simulink model "TailSitter_PX4"  (R2018b)
settings: Solver=VariableStepAuto  StartTime=0.0  StopTime=1100  RelTol=1e-3
values from neighbouring files (symbols this model uses):
  p =     [ds.mat]    (also in vxs.mat)
undefined symbols (not defined in the file or in its folder): quatnormalize
libraries: aerolibutil x24, simulink x14, sharedtransform x6, vrlib x4, sharedutil x3, simulink_extras x2, aerolibanim x1, aerolibanimutils x1
(part 2 of 3)

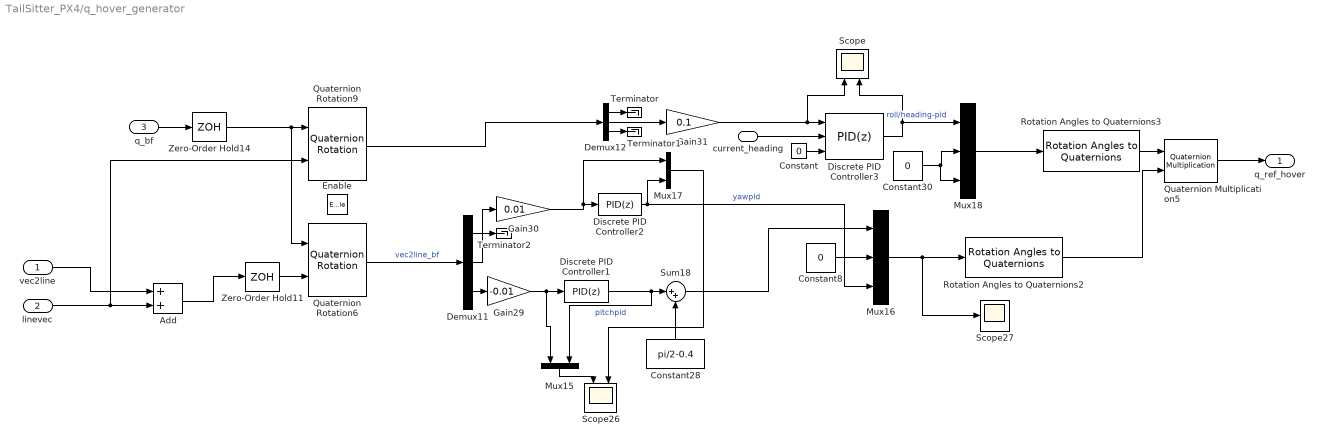
== system TailSitter_PX4/q_hover_generator ==
  vec2line : Inport
  linevec : Inport  Port=2
  q_bf : Inport  Port=3
  current_heading : Inport  Port=4
  Enable : EnablePort  StatesWhenEnabling=reset
  Add : Sum
  Constant : Constant  Value=0
  Constant28 : Constant  Value=pi/2-0.4
  Constant30 : Constant  Value=0
  Constant8 : Constant  Value=0
  Demux11 : Demux  Outputs=3
  Demux12 : Demux  Outputs=3
  Discrete PID Controller1 : simulink/Continuous/PID Controller  Controller=PID  Form=Parallel  TimeDomain=Discrete-time  SampleTime=-1  IntegratorMethod=Forward Euler  FilterMethod=Forward Euler  ControllerParametersSource=internal  P=0.75  I=0.1  D=8  UseFilter=off  N=100  TunerSelectOption=Transfer Function Based (PID Tuner App)  InitialConditionSource=internal  InitialConditionForIntegrator=0  InitialConditionForFilter=0  DifferentiatorICPrevScaledInput=0  ExternalReset=none  TrackingMode=off  Kt=1  LimitOutput=on  UpperSaturationLimit=deg2rad(40)  LowerSaturationLimit=-deg2rad(40)  LinearizeAsGain=off  AntiWindupMode=none  Kb=1  POutMin=[]  POutMax=[]  IOutMin=[]  IOutMax=[]  DOutMin=[]  DOutMax=[]  NOutMin=[]  NOutMax=[]  SumOutMin=[]  SumOutMax=[]  SaturationOutMin=[]  SaturationOutMax=[]  PParamMin=[]  PParamMax=[]  IParamMin=[]  IParamMax=[]  DParamMin=[]  DParamMax=[]  NParamMin=[]  NParamMax=[]  KbParamMin=[]  KbParamMax=[]  KtParamMin=[]  KtParamMax=[]  KbOutMin=[]  KbOutMax=[]  KtOutMin=[]  KtOutMax=[]  IntegratorOutMin=[]  IntegratorOutMax=[]  FilterOutMin=[]  FilterOutMax=[]  SumI1OutMin=[]  SumI1OutMax=[]  SumI2OutMin=[]  SumI2OutMax=[]  SumI3OutMin=[]  SumI3OutMax=[]  SumI4OutMin=[]  SumI4OutMax=[]  SumDOutMin=[]  SumDOutMax=[]  DifferentiatorOutMin=[]  DifferentiatorOutMax=[]  FilterDiffOutCoefMin=[]  FilterDiffOutCoefMax=[]  ReciprocalOutMin=[]  ReciprocalOutMax=[]  SumDenOutMin=[]  SumDenOutMax=[]  SumNumOutMin=[]  SumNumOutMax=[]  DivideOutMin=[]  DivideOutMax=[]  IntegratorContinuousStateAttributes=''  IntegratorStateMustResolveToSignalObject=off  IntegratorRTWStateStorageClass=Auto  FilterContinuousStateAttributes=''  FilterStateMustResolveToSignalObject=off  FilterRTWStateStorageClass=Auto  ParallelPVariant=InternalParameters  IdealPVariant=Disabled  IVariant=InternalParameters  DVariant=InternalParameters  IntegratorVariant=Discrete  SatVariant=Enabled  AWVariant=Passthrough  PCopyVariant=Disabled  TRVariant=Disabled  FdbkBlocksVariant=Forward  IdealPFdbkVariant=Disabled  SatFdbkVariant=Disabled  DerivativeFilterVariant=Differentiator  NVariant=Passthrough  NCopyVariant=Disabled_SignalSpec  FilterICVariant=InternalICsDifferentiator  IntegratorICVariant=InternalICs  ExternalResetVariant=Disabled  TRSumVariant=Passthrough  SumFdbkVariant=Disabled  SumVariant=Sum_PID
  Discrete PID Controller2 : simulink/Continuous/PID Controller  Controller=PID  Form=Parallel  TimeDomain=Discrete-time  SampleTime=-1  IntegratorMethod=Forward Euler  FilterMethod=Forward Euler  ControllerParametersSource=internal  P=1  I=0  D=2  UseFilter=off  N=100  TunerSelectOption=Transfer Function Based (PID Tuner App)  InitialConditionSource=internal  InitialConditionForIntegrator=0  InitialConditionForFilter=0  DifferentiatorICPrevScaledInput=0  ExternalReset=none  TrackingMode=off  Kt=1  LimitOutput=on  UpperSaturationLimit=deg2rad(40)  LowerSaturationLimit=-deg2rad(40)  LinearizeAsGain=off  AntiWindupMode=none  Kb=1  POutMin=[]  POutMax=[]  IOutMin=[]  IOutMax=[]  DOutMin=[]  DOutMax=[]  NOutMin=[]  NOutMax=[]  SumOutMin=[]  SumOutMax=[]  SaturationOutMin=[]  SaturationOutMax=[]  PParamMin=[]  PParamMax=[]  IParamMin=[]  IParamMax=[]  DParamMin=[]  DParamMax=[]  NParamMin=[]  NParamMax=[]  KbParamMin=[]  KbParamMax=[]  KtParamMin=[]  KtParamMax=[]  KbOutMin=[]  KbOutMax=[]  KtOutMin=[]  KtOutMax=[]  IntegratorOutMin=[]  IntegratorOutMax=[]  FilterOutMin=[]  FilterOutMax=[]  SumI1OutMin=[]  SumI1OutMax=[]  SumI2OutMin=[]  SumI2OutMax=[]  SumI3OutMin=[]  SumI3OutMax=[]  SumI4OutMin=[]  SumI4OutMax=[]  SumDOutMin=[]  SumDOutMax=[]  DifferentiatorOutMin=[]  DifferentiatorOutMax=[]  FilterDiffOutCoefMin=[]  FilterDiffOutCoefMax=[]  ReciprocalOutMin=[]  ReciprocalOutMax=[]  SumDenOutMin=[]  SumDenOutMax=[]  SumNumOutMin=[]  SumNumOutMax=[]  DivideOutMin=[]  DivideOutMax=[]  IntegratorContinuousStateAttributes=''  IntegratorStateMustResolveToSignalObject=off  IntegratorRTWStateStorageClass=Auto  FilterContinuousStateAttributes=''  FilterStateMustResolveToSignalObject=off  FilterRTWStateStorageClass=Auto  ParallelPVariant=InternalParameters  IdealPVariant=Disabled  IVariant=InternalParameters  DVariant=InternalParameters  IntegratorVariant=Discrete  SatVariant=Enabled  AWVariant=Passthrough  PCopyVariant=Disabled  TRVariant=Disabled  FdbkBlocksVariant=Forward  IdealPFdbkVariant=Disabled  SatFdbkVariant=Disabled  DerivativeFilterVariant=Differentiator  NVariant=Passthrough  NCopyVariant=Disabled_SignalSpec  FilterICVariant=InternalICsDifferentiator  IntegratorICVariant=InternalICs  ExternalResetVariant=Disabled  TRSumVariant=Passthrough  SumFdbkVariant=Disabled  SumVariant=Sum_PID
  Discrete PID Controller3 : simulink/Continuous/PID Controller  Controller=PID  Form=Parallel  TimeDomain=Discrete-time  SampleTime=-1  IntegratorMethod=Forward Euler  FilterMethod=Forward Euler  ControllerParametersSource=internal  P=1  I=1  D=0  UseFilter=off  N=100  TunerSelectOption=Transfer Function Based (PID Tuner App)  InitialConditionSource=external  InitialConditionForIntegrator=0  InitialConditionForFilter=0  DifferentiatorICPrevScaledInput=0  ExternalReset=none  TrackingMode=off  Kt=1  LimitOutput=off  UpperSaturationLimit=deg2rad(40)  LowerSaturationLimit=-deg2rad(40)  LinearizeAsGain=off  AntiWindupMode=none  Kb=1  POutMin=[]  POutMax=[]  IOutMin=[]  IOutMax=[]  DOutMin=[]  DOutMax=[]  NOutMin=[]  NOutMax=[]  SumOutMin=[]  SumOutMax=[]  SaturationOutMin=[]  SaturationOutMax=[]  PParamMin=[]  PParamMax=[]  IParamMin=[]  IParamMax=[]  DParamMin=[]  DParamMax=[]  NParamMin=[]  NParamMax=[]  KbParamMin=[]  KbParamMax=[]  KtParamMin=[]  KtParamMax=[]  KbOutMin=[]  KbOutMax=[]  KtOutMin=[]  KtOutMax=[]  IntegratorOutMin=[]  IntegratorOutMax=[]  FilterOutMin=[]  FilterOutMax=[]  SumI1OutMin=[]  SumI1OutMax=[]  SumI2OutMin=[]  SumI2OutMax=[]  SumI3OutMin=[]  SumI3OutMax=[]  SumI4OutMin=[]  SumI4OutMax=[]  SumDOutMin=[]  SumDOutMax=[]  DifferentiatorOutMin=[]  DifferentiatorOutMax=[]  FilterDiffOutCoefMin=[]  FilterDiffOutCoefMax=[]  ReciprocalOutMin=[]  ReciprocalOutMax=[]  SumDenOutMin=[]  SumDenOutMax=[]  SumNumOutMin=[]  SumNumOutMax=[]  DivideOutMin=[]  DivideOutMax=[]  IntegratorContinuousStateAttributes=''  IntegratorStateMustResolveToSignalObject=off  IntegratorRTWStateStorageClass=Auto  FilterContinuousStateAttributes=''  FilterStateMustResolveToSignalObject=off  FilterRTWStateStorageClass=Auto  ParallelPVariant=InternalParameters  IdealPVariant=Disabled  IVariant=InternalParameters  DVariant=InternalParameters  IntegratorVariant=Discrete  SatVariant=Disabled  AWVariant=Passthrough  PCopyVariant=Disabled  TRVariant=Disabled  FdbkBlocksVariant=Forward  IdealPFdbkVariant=Disabled  SatFdbkVariant=Disabled  DerivativeFilterVariant=Differentiator  NVariant=Passthrough  NCopyVariant=Disabled_SignalSpec  FilterICVariant=ExternalICs  IntegratorICVariant=ExternalICs  ExternalResetVariant=Disabled  TRSumVariant=Passthrough  SumFdbkVariant=Disabled  SumVariant=Sum_PID
  Gain29 : Gain  Gain=-0.01
  Gain30 : Gain  Gain=0.01
  Gain31 : Gain  Gain=0.1
  Mux15 : Mux  Inputs=2
  Mux16 : Mux  Inputs=3
  Mux17 : Mux  Inputs=2
  Mux18 : Mux  Inputs=3
  Quaternion Multiplication5 : aerolibutil/Quaternion Multiplication
  Quaternion Rotation6 : aerolibutil/Quaternion Rotation
  Quaternion Rotation9 : aerolibutil/Quaternion Rotation
  Rotation Angles to Quaternions2 : sharedtransform/Rotation Angles to Quaternions  rotationOrder=YXZ  aMode=aMode
      settings: SourceProductName=Aerospace Blockset  SourceProductBaseCode=AE
  Rotation Angles to Quaternions3 : sharedtransform/Rotation Angles to Quaternions  rotationOrder=ZYX  aMode=aMode
      settings: SourceProductName=Aerospace Blockset  SourceProductBaseCode=AE
  Scope : Scope  NumInputPorts=2
  Scope26 : Scope  NumInputPorts=2
  Scope27 : Scope
  Sum18 : Sum  Inputs=|++
  Terminator : Terminator
  Terminator1 : Terminator
  Terminator2 : Terminator
  Zero-Order Hold11 : ZeroOrderHold  SampleTime=p.Ts
  Zero-Order Hold14 : ZeroOrderHold  SampleTime=p.Ts
  q_ref_hover : Outport
  wires:
  vec2line/1 -> Add/1
  Discrete PID Controller1/1 -> Sum18/1, Mux15/2  "pitchpid"
  Gain29/1 -> Mux15/1, Discrete PID Controller1/1
  Demux11/2 -> Gain30/1
  Quaternion Rotation6/1 -> Demux11/1  "vec2line_bf"
  Constant30/1 -> Mux18/3, Mux18/2
  Demux12/3 -> Terminator1/1
  Demux12/1 -> Terminator/1
  Gain31/1 -> Scope/1, Discrete PID Controller3/1
  linevec/1 -> Quaternion Rotation9/2, Add/2
  Discrete PID Controller3/1 -> Scope/2, Mux18/1  "roll/heading-pid"
  Mux15/1 -> Scope26/1
  Mux16/1 -> Scope27/1, Rotation Angles to Quaternions2/1
  Rotation Angles to Quaternions3/1 -> Quaternion Multiplication5/1
  q_bf/1 -> Zero-Order Hold14/1
  Demux11/3 -> Gain29/1
  Constant8/1 -> Mux16/2
  Discrete PID Controller2/1 -> Mux16/3, Mux17/2  "yawpid"
  Rotation Angles to Quaternions2/1 -> Quaternion Multiplication5/2
  Mux18/1 -> Rotation Angles to Quaternions3/1
  Quaternion Multiplication5/1 -> q_ref_hover/1
  Demux12/2 -> Gain31/1
  Mux17/1 -> Scope26/2
  Add/1 -> Zero-Order Hold11/1
  Zero-Order Hold14/1 -> Quaternion Rotation6/1, Quaternion Rotation9/1
  Constant28/1 -> Sum18/2
  Gain30/1 -> Mux17/1, Discrete PID Controller2/1
  Zero-Order Hold11/1 -> Quaternion Rotation6/2
  Demux11/1 -> Terminator2/1
  Sum18/1 -> Mux16/1
  Constant/1 -> Discrete PID Controller3/3
  current_heading/1 -> Discrete PID Controller3/2
  Quaternion Rotation9/1 -> Demux12/1

== matlab function TailSitter_PX4/Torque_FL ==
  data: u_omegaL output; u_omegaR output; u_deltaL output; u_deltaR output; tao input; states input; u_jointT input; p parameter
function [u_omegaL,u_omegaR, u_deltaL,u_deltaR]  = FL_torques(tao, states, u_jointT, p)


wxr = tao(1); % I wonder if this comversion from omega to tao is right? Depends on Emil Fresk implementation
wyr = tao(2);
wzr = tao(3);
v = states(1:3);
vx = v(1);
vy = v(2);
vz = v(3);
w = states(4:6);
wx = w(1);
wy = w(2);
wz = w(3);
q = states(7:10); % Possibly not needed?
q0=q(1);
q1=q(2);
q2=q(3);
q3=(4);
deltaL = states(11);
deltaR = states(12);
omegaL = states(13);
omegaR = states(14);

% init output vector
u_deltaL = 0;
u_deltaR = 0;
u_omegaL = 0;
u_omegaR = 0;

% If you know of a better way (not counting modifying the code below to use
% p.x notation, plese feel welcome to tell me.
%P = struct2cell(p);
%Pn = fieldnames(p);
%for i=1:numel(P)
%    eval(Pn{i}+"="+string(P{i})+";")
%end
Ts=p.Ts;
m=p.m;
Ix=p.Ix;
Iy=p.Iy;
Iz=p.Iz;
I=p.I;
g=p.g;
rho=p.rho;
propd=p.propd;
K_T=p.K_T;
K_v=p.K_v;
b_w=p.b_w;
Sa=p.Sa;
Saw=p.Saw;
CLdelta=p.CLdelta;
CDdelta=p.CDdelta;
SW=p.SW;
Sw_w=p.Sw_w;
Sw=p.Sw;
b=p.b;
Cmyl=p.Cmyl;
Cwy=p.Cwy;
yf=p.yf;
yt=p.yt;
xW=p.xW;
xf=p.xf;
xac=p.xac;
zW=p.zW;
yw=p.yw;
yW=p.yW;
yWE=p.yWE;
yWEE=p.yWEE;
K_omegaL=p.K_omegaL;
K_omegaR=p.K_omegaR;
K_deltaL=p.K_deltaL;
K_deltaR=p.K_deltaR;
CL_A=p.CL_A;
CL_B=p.CL_B;
CL_C=p.CL_C;
CD_A=p.CD_A;
CD_B=p.CD_B;
CD_C=p.CD_C;
CLB_A=p.CLB_A;
CLB_B=p.CLB_B;
CDB_A=p.CDB_A;
CDB_B=p.CDB_B;
% The constants below are for the polynomial approximations.
% I am lookin into a way of auto-generating them in a struct or something.
a11=p.a11;
a12=p.a12;
a13=p.a13;
a21=p.a21;
a22=p.a22;
a23=p.a23;
a31=p.a31;
a32=p.a32;
a33=p.a33;
a41=p.a41;
a42=p.a42;
a43=p.a43;
b11=p.b11;
b12=p.b12;
b13=p.b13;
b14=p.b14;
b21=p.b21;
b22=p.b22;
b23=p.b23;
b24=p.b24;
b31=p.b31;
b32=p.b32;
b33=p.b33;
b34=p.b34;
c11=p.c11;
c12=p.c12;
c13=p.c13;
c14=p.c14;
c21=p.c21;
c22=p.c22;
c23=p.c23;
c24=p.c24;
c31=p.c31;
c32=p.c32;
c33=p.c33;
c34=p.c34;
c41=p.c41;
c42=p.c42;
c43=p.c43;
c44=p.c44;
% Assuming we made correct choices here it should suffice with this:
%u = [u_deltaA u_jointA u_deltaT]';


% Hey, anyone reading this? Code below is auto-generated because the
% F.L. was just too much of a headache to do
% manyally, so I wrote a script for it.
wn = p.wn;
u_ref =[ ...
];
 
u_deltaA = u_ref(1);
u_jointA = u_ref(2);
u_deltaT = u_ref(3);

u_deltaL = u_jointA - u_deltaA/2;
u_deltaR = u_jointA + u_deltaA/2;
u_omegaL = u_jointT + u_deltaT/2;
u_omegaR = u_jointT - u_deltaT/2;

gain = 1;
u_deltaL = gain*u_deltaL;
u_deltaR = gain*u_deltaR;

end

== matlab function TailSitter_PX4/TailSitter/tailsittersimv2 ==
  data: omegaLdot output; omegaRdot output; deltaLdot output; deltaRdot output; qdot output; wdot output; vdot output; omegaL input; omegaR input; deltaL input; deltaR input; u_omegaL input; u_omegaR input; u_deltaL input; u_deltaR input; q input; w input; v input; wind_v input; p parameter; alpha output; Beta output; g_out output
function [ omegaLdot, omegaRdot, deltaLdot, deltaRdot, qdot,wdot,vdot, alpha, Beta, g_out] = ...
    tailsitter_v2(omegaL, omegaR, deltaL, deltaR, u_omegaL, u_omegaR, u_deltaL, ...
    u_deltaR, q,w,v, wind_v, p)

% Set output port dim
omegaLdot = 0;
omegaRdot = 0;
deltaLdot = 0;
deltaRdot = 0;
alpha = 0;
Beta = 0;
qdot = zeros(4,1);
wdot = zeros(3,1);
vdot = zeros(3,1);
g_out = zeros(3,1);

% Map inputs
vx = v(1) + wind_v(1);
vy = v(2) + wind_v(2);
vz = v(3) + wind_v(3);

wx = w(1);
wy = w(2);
wz = w(3);

q0 = q(1);
q1 = q(2);
q2 = q(3);
q3 = q(4);

% function handles not supported, so adding here directly
c = @(y) 0.28 - (0.28-0.09).*abs(y)./(p.b/2); % This should be pretty accurate
% Lift curves
CL = @(alpha) p.CL_A*sin(p.CL_B.*alpha)+p.CL_C; % These are wrong, just placeholders
CD = @(alpha) p.CD_A-p.CD_A.*cos(p.CD_B.*alpha)+p.CD_C;

alpha = atan2(vz,vx);

%Thrust
TL = p.K_T .* omegaL.^2;
TR = p.K_T .* omegaR.^2;

% airflow in thrust wake
v_w_L = p.b_w .* omegaL; %[b_w .* omegaL; vy; vz];
v_w_R = p.b_w .* omegaR;
%alpha_wL = atan2(vz,v_w_L);
%alpha_wR = atan2(vz,v_w_R);

% Quaternion
qdot = 0.5.*[-q1 -q2 -q3; ...
            q0 -q3 q2; ...
            q3 q0 -q1; ...
            -q2 q1 q0]*w;

% inputs
deltaLdot = p.K_deltaL .* (-deltaL + u_deltaL);
deltaRdot = p.K_deltaR .* (-deltaR + u_deltaR);
omegaLdot = p.K_omegaL .* (-omegaL + u_omegaL);
omegaRdot = p.K_omegaR .* (-omegaR + u_omegaR);

% gravity
% To get vector g in bf from wf
% we need to rotate it by q_wf, or conj(q_bf)
qc = quatconj([q0 q1 q2 q3]); %
qc0 = qc(1);
qc1 = qc(2);
qc2 = qc(3);
qc3 = qc(4);
gravity = p.g .* [2.*(qc1.*qc3 + qc0.*qc2); ...
                2.*(qc2.*qc3 - qc0.*qc1); ...
                (qc0.^2 - qc1.^2 - qc2.^2 + qc3.^2);
                zeros(3+4+4,1)];
g_out = gravity(1:3,1);
% Inertial forces
inertialF = -[2*(vz.*wy - vy.*wz); ...
             2*(vx.*wz - vz.*wx); ...
             2*(vy.*wx - vx.*wy); ...
             (p.Iz - p.Iy).*wy.*wz./p.Ix; ...
             (p.Ix - p.Iz).*wx.*wz./p.Iy; ...
             (p.Iy - p.Ix).*wx.*wy./p.Iz; ...
             zeros(8,1)];
%Sideslip
Beta = atan2(vy,vx);

% Winglets
CLB = @(beta) p.CLB_A*sin(p.CLB_B.*beta); % These are wrong, just placeholders
CDB = @(beta) p.CDB_A-p.CDB_A.*cos(p.CDB_B.*beta);
L_W = -p.rho * sqrt(vx.^2+vy.^2) * p.SW * (CLB(Beta)*vx + CDB(Beta)*vy); % Lift in bodyframe, y
D_W = p.rho * sqrt(vx.^2+vy.^2) * p.SW * (-CLB(Beta)*vy + CDB(Beta)*vx); % Drag in bodyfram, x

% MAIN WING
% Lift inside wake
LLT = p.Sw_w * 0.5 * p.rho * abs(v_w_L) .* CL(0).*v_w_L ;
LRT = p.Sw_w * 0.5 * p.rho * abs(v_w_R) .* CL(0).*v_w_R ;
% Lift outside wake
LL = p.Sw * 0.5 * p.rho * sqrt(vx.^2 + vz.^2) .* ...
    (CL(alpha).*vx + CD(alpha).*vz);
LR = LL; % Yeah we -could- combine these, but too late!
% Drag inside wake
DLT = p.Sw_w * 0.5 * p.rho * abs(v_w_L) * CD(0) * v_w_L;
DRT = p.Sw_w * 0.5 * p.rho * abs(v_w_R) * CD(0) * v_w_R;
% Drag outside wake
DL = p.Sw * 0.5 * p.rho * sqrt(vx.^2  + vz.^2) .* ...
    (-CL(alpha).*vz + CD(alpha).*vx);
DR = DL; % Yeah, we -could- combine these as well...

% AILERONS
% Lift inside wake, signs bc rotation dir of aileron
FLT = -p.CLdelta * 0.5*p.rho*v_w_L.^2 * p.Saw * deltaL;
FRT = -p.CLdelta * 0.5*p.rho*v_w_R.^2 * p.Saw * deltaR;
% Lift outside wake
FL = -sign(vx).*p.CLdelta * 0.5*p.rho*(vx.^2 + vy.^2 + vz.^2) * p.Sa * deltaL;
FR = -sign(vx).*p.CLdelta * 0.5*p.rho*(vx.^2 + vy.^2 + vz.^2) * p.Sa * deltaR;
% Drag inside wake
DalphaLT =p.CDdelta * 0.5*p.rho*v_w_L.^2 * p.Saw * abs(deltaL);
DalphaRT = p.CDdelta * 0.5*p.rho*v_w_R.^2 * p.Saw * abs(deltaR);
% Drag outside wake, we add sign of vx because we might be reversing?
DalphaL = sign(vx).*p.CDdelta * 0.5*p.rho*(vx.^2 + vy.^2 + vz.^2) * p.Sa * abs(deltaL);
DalphaR = sign(vx).*p.CDdelta * 0.5*p.rho*(vx.^2 + vy.^2 + vz.^2) * p.Sa * abs(deltaR);

% f1
 % diff in ail deflection
  % inside wake
  % outside wake
 % resmom roll,
 % roll due to yaw rate
 % moment due to sideslip
alphal_rmr = @(y) atan2(vz+wx.*y, vx);
restmomroll = @(y) y .* c(y) .* sqrt(vx.^2 + (vz+wx.*y).^2) .* ...
    (CL(alphal_rmr(y)).*vx + CD(alphal_rmr(y)).*(vz+wx.*y));
alphal_rwz = @(y) atan2(vz, vx-wz.*y);
rollduetowz = @(y) y .* c(y) .* sqrt((vx-wz.*y).^2 + vz.^2) .* ...
    (CL(alphal_rwz(y)).*(vx-wz*y) + CD(alphal_rwz(y)).*vz);
f1 = p.yf.*(FLT+FL -FRT-FR) ...
    -0.5*p.rho.*quadgk(restmomroll,-p.yW,p.yW) ... % between wakes
     -0.5*p.rho.*quadgk(restmomroll,-p.yWEE,-p.yWE) ... % outside left wake
      -0.5*p.rho.*quadgk(restmomroll,p.yWE,p.yWEE) ... % outside right wake
    -0.5*p.rho.*quadgk(rollduetowz,-p.yW,p.yW) ... between wakes
     -0.5*p.rho.*quadgk(rollduetowz,-p.yWEE,-p.yWE) ... left side
      -0.5*p.rho.*quadgk(rollduetowz, p.yWE,p.yWEE) ... right side
    +p.zW*L_W;
% f2
 % joint ail deflection
  % inside wake
  % outside wake
 % pitch moment
 % restmom pitch rate, --- compensate for wake!
 % Pitch from winglets
f2 = p.xf.*(FLT+FL+FRT+FR) ...
    ... %+ 0.5*p.rho*p.Cmyl*(2*p.Sw.*(vx.^2+vy.^2+vz.^2)+p.Sw_w*(v_w_L.^2 + v_w_R.^2) ) ...
    -p.xac.*(LL+LR+LLT+LRT) ... % We do not assume Pith coeff static.
    -wy.*p.rho.*2.*p.Sw.*p.Cwy.*sqrt(vx.^2 + vz.^2) ...
    +p.zW*D_W;
% f3
 % diff in T
 % mom due to sideslip
 % restmom yaw rate, compensate for outside wake
restmomwz = @(y) y .* c(y) .* sqrt((vx-wz.*y).^2 + vz.^2) .* ...
    (-CL(alphal_rwz(y)).*vz + CD(alphal_rwz(y)).*(vx-wz.*y));
f3 = p.yt.*(TL-TR) ...
     -p.xW*L_W ...
     +0.5*quadgk(restmomwz,-p.yW,p.yW) ...
     +0.5*quadgk(restmomwz,-p.yWEE,-p.yWE) ...
     +0.5*quadgk(restmomwz, p.yWE,p.yWEE);
 
%velocities
vxdot = (TL +TR -DL -DR -DLT -DRT -D_W -DalphaL -DalphaR -DalphaLT -DalphaRT)./p.m;
vydot = L_W./p.m;
vzdot = (-LL -LR -LLT -LRT +FL +FR +FLT +FRT)./p.m;

% angular rates
wxdot = f1./p.Ix;
wydot = f2./p.Iy;
wzdot = f3./p.Iz;

%if any(abs(vxdot) > 100)
%    p.m
%end

statesdot = gravity + inertialF +  ...
    [vxdot;vydot;vzdot;wxdot;wydot;wzdot;qdot;...
    deltaLdot;deltaRdot;omegaLdot;omegaRdot];

vdot = statesdot(1:3);
wdot = statesdot(4:6);
qdot = statesdot(7:10);
deltaLdot = statesdot(11);
deltaRdot = statesdot(12);
omegaLdot = statesdot(13);
omegaRdot = statesdot(14);

== matlab function TailSitter_PX4/TailSitter/myQuatNorm ==
  data: q input; n output
function n = fcn(q)

n = sqrt(q(1).^2 + q(2).^2 + q(3).^2 + q(4).^2);

== matlab function TailSitter_PX4/MATLAB Function ==
  data: u input; y output
function y = norm(u)

y = sqrt(sum(u.^2));

== matlab function TailSitter_PX4/TailSitter/MATLAB Function ==
  data: time input; w output
function w = rotsteps(time)

stept = 10;
wt = 10;
reverse = 0;
if time<stept
    w = [0.1,0,0];
elseif time<stept+wt
    if reverse
        w = [-0.1,0,0];
    else
        w = zeros(1,3);
    end
elseif time<2*stept+wt
    w = [0,0,0.1];
elseif time<2*stept+2*wt
    if reverse
        w = [0,0,-0.1];
    else
        w = zeros(1,3);
    end
else
    w = [0,0.1,0];
end

== matlab function TailSitter_PX4/MATLAB Function2 ==
  data: q_wf input; q_ref output
function q_ref = refquat(q_wf)

% TODO: Figure out how to set a good reference quaternion.
q_ref = q_wf;

== matlab function TailSitter_PX4/MATLAB Function1 ==
  data: v_ref input; q_ref output; u_jointT output
function [q_ref,u_jointT] = ref_quat(v_ref)


q_ref = [1,0,0,0]';
u_jointT = 300;

% We have output of 5dof.
% Input is 3dof.
% We can extend input dof by saying we want wings to be horizontal, now
% total in is 4dof.


%Construct quaterion from several different rotations?

== matlab function TailSitter_PX4/linegenerator ==
  settings: updateMethod=DISCRETE
  data: v_wf input; r input; p parameter; rspeed output; wpN output; dist2wp output; linevec output; vec2line output; wp_r output
function [rspeed,wpN, dist2wp, linevec, vec2line, wp_r] = LineGenerator( v_wf,r, p)

% Keep track of which waypoint we are going to
persistent waypointno;
persistent wp;
persistent wp_prev;
persistent miss;
if isempty(waypointno)
    waypointno=2;
    wp=p.waypoints(waypointno,:)';
    wp_prev=p.waypoints(waypointno-1,:)';
    miss=0;
end

%initialize variables
dist2line2d = 0;
altError = 0;
thetaerr = 0;
rspeed = 0;
vec2line = [0,0,0]';

% if current waypoint is the start wp/home wp jump immediately to next.
dist2wp = sqrt( sum( (wp(1:3)-r).^2 ) );
if dist2wp <= wp(5)
    if waypointno < p.numwp
        waypointno = waypointno+1;
    else
        waypointno = 2; % we always skip home wp at origin
    end
    wp_prev = wp;
    wp = p.waypoints(waypointno,:)';
    miss=0;
end
rspeed = wp(4);
wp_r = wp(1:3); % Next waypoint position, v has been scaled away thus wp_r

% find vector between last waypoint and current target
linevec = (wp(1:3)-wp_prev(1:3))./sqrt( sum((wp(1:3)-wp_prev(1:3)).^2) );

% Check if we missed our goal!
%{
if ~miss && dot(linevec, wp(1:3)-r) < 0 && sqrt(sum( (wp(1:3)-r).^2 )) > wp(5)*2
    linevec(1:2)=-linevec(1:2);
    miss=1;
elseif miss
    linevec(1:2)=-linevec(1:2);
end
%}
if  dot(linevec, wp(1:3)-r) < 0 
    linevec(1:3)=-linevec(1:3);
end
% Figure out if goal is ahead of us or if we passed it/missed it.
%if dot(v_wf(1:3), wp(1:3)-r(1:3)) < 0
%    linevec(1:2) = - linevec(1:2);
%end
% THe above doesn't work.

%{
% find angle in x-y plane of vector
thetastar = atan2(linevec(2), linevec(1));
% find our current heading
theta = atan2(v_wf(2),v_wf(1));
% Error in direction along line / be paralell with line
thetaerr = thetastar - theta;
%}

% Find the vector that describes the vector to the closest point on the
% line
a = wp_prev(1:3);               % Points to "start of line"
n = linevec;                    % Points toward next wp
vec2line = a-r - dot(a-r,n)*n;
%altError = vec2line(3);
%dist2line2d = sqrt( sum( vec2line(1:2).^2 ));
wpN = waypointno;


% Mix the vectors for reference according to how far away from line we are

% Old setup, constants: 0.0075/0.01, max/dl2coeff
%{
%cr = cross(linevec,vec2line);
%refvec = linevec;
vcomp = (12/rspeed).^2;
if abs(d2lcoeff*dist2line2d) < max2l*vcomp
    refvec = linevec + d2lcoeff*dist2line2d*vec2line;
else
    refvec = linevec + vcomp*max2l*vec2line;
end
}
%}

%{
vcomp=1/rspeed;
refvec = linevec+vec2line*d2lcoeff*vcomp;

refvec = refvec/sqrt(sum(refvec.^2));
%}

== matlab function TailSitter_PX4/AdHoc1 ==
  data: u_jointT input; states input; u_omegaL output; u_omegaR output; u_deltaL output; u_deltaR output; tx input; ty input; tz input; cond_M output; p parameter
function [u_omegaL,u_omegaR, u_deltaL,u_deltaR, cond_M]  = AdHocTorques( u_jointT, states, tx, ty, tz, p)

% This is a crude/simple input/output/actuator linker.
% A pitch torque is made by moving elevons in the same direction: jointA.
% A roll torque is made by moving elevons in opposite direction: deltaA.
% A yaw torque is made by a differential thrust of the engines: deltaT.
% Power forward is given and passed straight through this function as
% jointT.

u_deltaL = 0;
u_deltaR = 0;
u_omegaL = 0;
u_omegaR = 0;
cond_M = 0;

wxr = -tx;
wyr = -ty;
wzr = -tz;

v = states(1:3);
vx = v(1);
vy = v(2);
vz = v(3);
w = states(4:6);
wx = w(1);
wy = w(2);
wz = w(3);
q = states(7:10); % Possibly not needed?
q0=q(1);
q1=q(2);
q2=q(3);
q3=q(4);
deltaL = states(11);
deltaR = states(12);
omegaL = states(13);
omegaR = states(14);
a11=p.a11;
a12=p.a12;
a13=p.a13;
a21=p.a21;
a22=p.a22;
a23=p.a23;
a31=p.a31;
a32=p.a32;
a33=p.a33;
a41=p.a41;
a42=p.a42;
a43=p.a43;
b11=p.b11;
b12=p.b12;
b13=p.b13;
b14=p.b14;
b21=p.b21;
b22=p.b22;
b23=p.b23;
b24=p.b24;
b31=p.b31;
b32=p.b32;
b33=p.b33;
b34=p.b34;
c11=p.c11;
c12=p.c12;
c13=p.c13;
c14=p.c14;
c21=p.c21;
c22=p.c22;
c23=p.c23;
c24=p.c24;
c31=p.c31;
c32=p.c32;
c33=p.c33;
c34=p.c34;
c41=p.c41;
c42=p.c42;
c43=p.c43;
c44=p.c44;
wn = 1;

M = [ ...
0.504*sign(vx)*(vx^2 + vy^2 + vz^2) + 0.0002901*omegaL^2 + 0.0002901*omegaR^2,                                       0.0005803*omegaR^2 - 0.0005803*omegaL^2,                                                                                                                                                                                                                                                        - 0.001161*deltaL*omegaL - 0.001161*deltaR*omegaR;
                                         0.001526*omegaL^2 - 0.001526*omegaR^2, - 0.003053*omegaL^2 - 0.003053*omegaR^2 - 5.303*sign(vx)*(vx^2 + vy^2 + vz^2), -(3.732e-21*(7.232e16*omegaL*sign(omegaR) - 7.232e16*omegaR*sign(omegaL) + 7.232e16*omegaL*sign(omegaL)^2*sign(omegaR) - 7.232e16*omegaR*sign(omegaL)*sign(omegaR)^2 + 1.636e18*deltaL*omegaL*sign(omegaL)*sign(omegaR) - 1.636e18*deltaR*omegaR*sign(omegaL)*sign(omegaR)))/(sign(omegaL)*sign(omegaR));
                                                                             0,                                                                             0,                                                                                                                                                                                                                                                                        0.002515*omegaL + 0.002515*omegaR ...
];
 
%Alpha/etc
K = [ ...
(14.29*wz*(b32*vx^2 + b22*vx + b12) + 14.29*wx*(a42*vx^3 + a32*vx^2 + a22*vx + a12) - 0.1008*deltaL*vz*sign(vx) + 0.1008*deltaR*vz*sign(vx) + 42.86*vz^2*wz*(b34*vx^2 + b24*vx + b14) + 28.57*vz*wx*(a43*vx^3 + a33*vx^2 + a23*vx + a13) + 28.57*vz*wz*(b33*vx^2 + b23*vx + b13))*(2.0*vy*wx - 2.0*vx*wy - 0.06827*(vx^2 + vz^2)^(1/2)*(vz*(2.0*cos(2.0*atan2(1.0*vz, vx)) - 2.05) - 1.0*vx*(1.2*sin(2.0*atan2(1.0*vz, vx)) + 0.2)) + 8.462e-6*deltaL*omegaL^2 + 8.462e-6*deltaR*omegaR^2 + 7.108e-6*omegaL*abs(omegaL) + 7.108e-6*omegaR*abs(omegaR) - 9.82*q0^2 + 9.82*q1^2 + 9.82*q2^2 - 9.82*q3^2 + 0.00735*deltaL*sign(vx)*(vx^2 + vy^2 + vz^2) + 0.00735*deltaR*sign(vx)*(vx^2 + vy^2 + vz^2)) - 1.03*wz*(0.06451*(vx^2 + vy^2)^(1/2)*(1.2*vy*sin(2.0*atan2(1.0*vy, vx)) + vx*(2.0*cos(2.0*atan2(1.0*vy, vx)) - 2.0)) + 25.93*wy*(vx^2 + vz^2)^(1/2) - 1.266*wx*wz - 0.2593*(vx^2 + vz^2)^(1/2)*(vz*(2.0*cos(2.0*atan2(1.0*vz, vx)) - 2.05) - 1.0*vx*(1.2*sin(2.0*atan2(1.0*vz, vx)) + 0.2)) + 0.0003053*deltaL*omegaL^2 + 0.0003053*deltaR*omegaR^2 + 2.699e-5*omegaL*abs(omegaL) + 2.699e-5*omegaR*abs(omegaR) + 0.2652*deltaL*sign(vx)*(vx^2 + vy^2 + vz^2) + 0.2652*deltaR*sign(vx)*(vx^2 + vy^2 + vz^2)) + 2.0*wn*(14.29*vz*(b32*wz*vx^2 + b22*wz*vx + b12*wz) - 0.00728*(vx^2 + vy^2)^(1/2)*(1.2*vx*sin(2.0*atan2(1.0*vy, vx)) - vy*(2.0*cos(2.0*atan2(1.0*vy, vx)) - 2.0)) + 14.29*vz*(a42*wx*vx^3 + a32*wx*vx^2 + a22*wx*vx + a12*wx) + 14.29*a11*wx + 14.29*b11*wz + 14.29*vz^2*(b33*wz*vx^2 + b23*wz*vx + b13*wz) + 14.29*vz^3*(b34*wz*vx^2 + b24*wz*vx + b14*wz) - 5.803e-5*deltaL*omegaL^2 + 5.803e-5*deltaR*omegaR^2 + 14.29*vz^2*(a43*wx*vx^3 + a33*wx*vx^2 + a23*wx*vx + a13*wx) + 14.29*a31*vx^2*wx + 14.29*a41*vx^3*wx + 14.29*b31*vx^2*wz - 0.0504*deltaL*sign(vx)*(vx^2 + vy^2 + vz^2) + 0.0504*deltaR*sign(vx)*(vx^2 + vy^2 + vz^2) + 14.29*a21*vx*wx + 14.29*b21*vx*wz) + (0.00728*(vx^2 + vy^2)^(1/2)*(2.0 + (2.4*vx^2*cos(2.0*atan2(1.0*vy, vx)))/(vx^2 + vy^2) + (4.0*vx*vy*sin(2.0*atan2(1.0*vy, vx)))/(vx^2 + vy^2) - 2.0*cos(2.0*atan2(1.0*vy, vx))) + 0.1008*deltaL*vy*sign(vx) - 0.1008*deltaR*vy*sign(vx) + (0.00728*vy*(2.0*vy - 2.0*vy*cos(2.0*atan2(1.0*vy, vx)) + 1.2*vx*sin(2.0*atan2(1.0*vy, vx))))/(vx^2 + vy^2)^(1/2))*(19.64*q0*q1 - 0.01699*(vx^2 + vy^2)^(1/2)*(1.2*vx*sin(2.0*atan2(1.0*vy, vx)) - vy*(2.0*cos(2.0*atan2(1.0*vy, vx)) - 2.0)) + 19.64*q2*q3 - 2.0*vx*wz + 2.0*vz*wx) - 10.0*deltaL*(0.0504*sign(vx)*(vx^2 + vy^2 + vz^2) + 5.803e-5*omegaL^2) + 10.0*deltaR*(0.0504*sign(vx)*(vx^2 + vy^2 + vz^2) + 5.803e-5*omegaR^2) - 1.0*(14.29*a11 + 14.29*a21*vx + 14.29*vz^2*(a43*vx^3 + a33*vx^2 + a23*vx + a13) + 14.29*a31*vx^2 + 14.29*a41*vx^3 + 14.29*vz*(a42*vx^3 + a32*vx^2 + a22*vx + a12))*(14.29*a11*wx - 0.00728*(vx^2 + vy^2)^(1/2)*(2.0*vy - 2.0*vy*cos(2.0*atan2(1.0*vy, vx)) + 1.2*vx*sin(2.0*atan2(1.0*vy, vx))) + 14.29*b11*wz - 1.03*wy*wz - 5.803e-5*deltaL*omegaL^2 + 5.803e-5*deltaR*omegaR^2 + 14.29*a31*vx^2*wx + 14.29*a41*vx^3*wx + 14.29*b31*vx^2*wz + 14.29*vz^2*wz*(b33*vx^2 + b23*vx + b13) + 14.29*vz^3*wz*(b34*vx^2 + b24*vx + b14) + 14.29*vz*wx*(a42*vx^3 + a32*vx^2 + a22*vx + a12) - 0.0504*deltaL*sign(vx)*(vx^2 + vy^2 + vz^2) + 0.0504*deltaR*sign(vx)*(vx^2 + vy^2 + vz^2) + 14.29*a21*vx*wx + 14.29*b21*vx*wz + 14.29*vz^2*wx*(a43*vx^3 + a33*vx^2 + a23*vx + a13) + 14.29*vz*wz*(b32*vx^2 + b22*vx + b12)) - 1.0*(14.29*b11 - 1.03*wy + 14.29*b21*vx + 14.29*vz*(b32*vx^2 + b22*vx + b12) + 14.29*b31*vx^2 + 14.29*vz^2*(b33*vx^2 + b23*vx + b13) + 14.29*vz^3*(b34*vx^2 + b24*vx + b14))*(0.05733*(vx^2 + vy^2)^(1/2)*(2.0*vy - 2.0*vy*cos(2.0*atan2(1.0*vy, vx)) + 1.2*vx*sin(2.0*atan2(1.0*vy, vx))) + 12.5*c11*wz + 0.7763*wx*wy + 0.0001258*omegaL^2 - 0.0001258*omegaR^2 + 12.5*c31*vx^2*wz + 12.5*c41*vx^3*wz + 12.5*vz*wz*(c42*vx^3 + c32*vx^2 + c22*vx + c12) + 12.5*c21*vx*wz + 12.5*vz^2*wz*(c43*vx^3 + c33*vx^2 + c23*vx + c13) + 12.5*vz^3*wz*(c44*vx^3 + c34*vx^2 + c24*vx + c14)) + wn^2*wx + wn^2*wxr + (19.64*q0*q2 - 0.06827*(vx^2 + vz^2)^(1/2)*(vx*(2.0*cos(2.0*atan2(1.0*vz, vx)) - 2.05) + vz*(1.2*sin(2.0*atan2(1.0*vz, vx)) + 0.2)) - 0.01699*(vx^2 + vy^2)^(1/2)*(1.2*vy*sin(2.0*atan2(1.0*vy, vx)) + vx*(2.0*cos(2.0*atan2(1.0*vy, vx)) - 2.0)) - 19.64*q1*q3 - 2.0*vy*wz + 2.0*vz*wy + 1.777e-6*omegaL*abs(omegaL) + 1.777e-6*omegaR*abs(omegaR) - 2.033e-5*omegaL^2 - 2.033e-5*omegaR^2 + 4.231e-7*omegaL^2*abs(deltaL) + 4.231e-7*omegaR^2*abs(deltaR) + 0.0003675*abs(deltaL)*sign(vx)*(vx^2 + vy^2 + vz^2) + 0.0003675*abs(deltaR)*sign(vx)*(vx^2 + vy^2 + vz^2))*(14.29*a21*wx + 14.29*b21*wz + 0.00728*(vx^2 + vy^2)^(1/2)*(- 1.2*sin(2.0*atan2(1.0*vy, vx)) + (4.0*vy^2*sin(2.0*atan2(1.0*vy, vx)))/(vx^2 + vy^2) + (2.4*vx*vy*cos(2.0*atan2(1.0*vy, vx)))/(vx^2 + vy^2)) + 42.86*a41*vx^2*wx - 0.1008*deltaL*vx*sign(vx) + 0.1008*deltaR*vx*sign(vx) + 14.29*vz*wx*(3.0*a42*vx^2 + 2.0*a32*vx + a22)  + 14.29*vz*wz*(b22 + 2.0*b32*vx) - (0.00728*vx*(2.0*vy - 2.0*vy*cos(2.0*atan2(1.0*vy, vx)) + 1.2*vx*sin(2.0*atan2(1.0*vy, vx))))/(vx^2 + vy^2)^(1/2) + 28.57*a31*vx*wx + 28.57*b31*vx*wz + 14.29*vz^2*wx*(3.0*a43*vx^2 + 2.0*a33*vx + a23) + 14.29*vz^2*wz*(b23 + 2.0*b33*vx) + 14.29*vz^3*wz*(b24 + 2.0*b34*vx)) - 0.0001161*deltaL*omegaL*(20.0*omegaL - 20.0*u_jointT) + 0.0001161*deltaR*omegaR*(20.0*omegaR - 20.0*u_jointT);
                                                                                                                                                                              wn^2*wy - 10.0*deltaL*(0.2652*sign(vx)*(vx^2 + vy^2 + vz^2) + 0.0003053*omegaL^2) - 10.0*deltaR*(0.2652*sign(vx)*(vx^2 + vy^2 + vz^2) + 0.0003053*omegaR^2) - 1.0*(0.2593*(vx^2 + vz^2)^(1/2)*(2.05 + (2.4*vx^2*cos(2.0*atan2(1.0*vz, vx)))/(vx^2 + vz^2) + (4.0*vx*vz*sin(2.0*atan2(1.0*vz, vx)))/(vx^2 + vz^2) - 2.0*cos(2.0*atan2(1.0*vz, vx))) + 0.5303*deltaL*vz*sign(vx) + 0.5303*deltaR*vz*sign(vx) + (25.93*vz*wy)/(vx^2 + vz^2)^(1/2) - (0.2593*vz*(vz*(2.0*cos(2.0*atan2(1.0*vz, vx)) - 2.05) - 1.0*vx*(1.2*sin(2.0*atan2(1.0*vz, vx)) + 0.2)))/(vx^2 + vz^2)^(1/2))*(2.0*vy*wx - 2.0*vx*wy - 0.06827*(vx^2 + vz^2)^(1/2)*(vz*(2.0*cos(2.0*atan2(1.0*vz, vx)) - 2.05) - 1.0*vx*(1.2*sin(2.0*atan2(1.0*vz, vx)) + 0.2)) + 8.462e-6*deltaL*omegaL^2 + 8.462e-6*deltaR*omegaR^2 + 7.108e-6*omegaL*abs(omegaL) + 7.108e-6*omegaR*abs(omegaR) - 9.82*q0^2 + 9.82*q1^2 + 9.82*q2^2 - 9.82*q3^2 + 0.00735*deltaL*sign(vx)*(vx^2 + vy^2 + vz^2) + 0.00735*deltaR*sign(vx)*(vx^2 + vy^2 + vz^2)) + (0.06451*(vx^2 + vy^2)^(1/2)*(1.2*sin(2.0*atan2(1.0*vy, vx)) - (4.0*vx^2*sin(2.0*atan2(1.0*vy, vx)))/(vx^2 + vy^2) + (2.4*vx*vy*cos(2.0*atan2(1.0*vy, vx)))/(vx^2 + vy^2)) + 0.5303*deltaL*vy*sign(vx) + 0.5303*deltaR*vy*sign(vx) + (0.06451*vy*(1.2*vy*sin(2.0*atan2(1.0*vy, vx)) + vx*(2.0*cos(2.0*atan2(1.0*vy, vx)) - 2.0)))/(vx^2 + vy^2)^(1/2))*(19.64*q0*q1 - 0.01699*(vx^2 + vy^2)^(1/2)*(1.2*vx*sin(2.0*atan2(1.0*vy, vx)) - vy*(2.0*cos(2.0*atan2(1.0*vy, vx)) - 2.0)) + 19.64*q2*q3 - 2.0*vx*wz + 2.0*vz*wx) - 1.266*wx*(0.05733*(vx^2 + vy^2)^(1/2)*(2.0*vy - 2.0*vy*cos(2.0*atan2(1.0*vy, vx)) + 1.2*vx*sin(2.0*atan2(1.0*vy, vx))) + 12.5*c11*wz + 0.7763*wx*wy + 0.0001258*omegaL^2 - 0.0001258*omegaR^2 + 12.5*c31*vx^2*wz + 12.5*c41*vx^3*wz + 12.5*vz*wz*(c42*vx^3 + c32*vx^2 + c22*vx + c12) + 12.5*c21*vx*wz + 12.5*vz^2*wz*(c43*vx^3 + c33*vx^2 + c23*vx + c13) + 12.5*vz^3*wz*(c44*vx^3 + c34*vx^2 + c24*vx + c14)) - 1.266*wz*(14.29*a11*wx - 0.00728*(vx^2 + vy^2)^(1/2)*(2.0*vy - 2.0*vy*cos(2.0*atan2(1.0*vy, vx)) + 1.2*vx*sin(2.0*atan2(1.0*vy, vx))) + 14.29*b11*wz - 1.03*wy*wz - 5.803e-5*deltaL*omegaL^2 + 5.803e-5*deltaR*omegaR^2 + 14.29*a31*vx^2*wx + 14.29*a41*vx^3*wx + 14.29*b31*vx^2*wz + 14.29*vz^2*wz*(b33*vx^2 + b23*vx + b13) + 14.29*vz^3*wz*(b34*vx^2 + b24*vx + b14) + 14.29*vz*wx*(a42*vx^3 + a32*vx^2 + a22*vx + a12) - 0.0504*deltaL*sign(vx)*(vx^2 + vy^2 + vz^2) + 0.0504*deltaR*sign(vx)*(vx^2 + vy^2 + vz^2) + 14.29*a21*vx*wx + 14.29*b21*vx*wz + 14.29*vz^2*wx*(a43*vx^3 + a33*vx^2 + a23*vx + a13) + 14.29*vz*wz*(b32*vx^2 + b22*vx + b12)) - 2.0*wn*(0.06451*(vx^2 + vy^2)^(1/2)*(1.2*vy*sin(2.0*atan2(1.0*vy, vx)) + vx*(2.0*cos(2.0*atan2(1.0*vy, vx)) - 2.0)) + 25.93*wy*(vx^2 + vz^2)^(1/2) - 0.2593*(vx^2 + vz^2)^(1/2)*(vz*(2.0*cos(2.0*atan2(1.0*vz, vx)) - 2.05) - 1.0*vx*(1.2*sin(2.0*atan2(1.0*vz, vx)) + 0.2)) + 0.0003053*deltaL*omegaL^2 + 0.0003053*deltaR*omegaR^2 + 2.699e-5*omegaL*abs(omegaL) + 2.699e-5*omegaR*abs(omegaR) + 0.2652*deltaL*sign(vx)*(vx^2 + vy^2 + vz^2) + 0.2652*deltaR*sign(vx)*(vx^2 + vy^2 + vz^2)) - 1.0*(20.0*omegaL - 20.0*u_jointT)*(2.699e-5*abs(omegaL) + 0.0006106*deltaL*omegaL + 2.699e-5*omegaL*sign(omegaL)) - 1.0*(20.0*omegaR - 20.0*u_jointT)*(2.699e-5*abs(omegaR) + 0.0006106*deltaR*omegaR + 2.699e-5*omegaR*sign(omegaR)) - 25.93*(vx^2 + vz^2)^(1/2)*(0.06451*(vx^2 + vy^2)^(1/2)*(1.2*vy*sin(2.0*atan2(1.0*vy, vx)) + vx*(2.0*cos(2.0*atan2(1.0*vy, vx)) - 2.0)) + 25.93*wy*(vx^2 + vz^2)^(1/2) - 1.266*wx*wz - 0.2593*(vx^2 + vz^2)^(1/2)*(vz*(2.0*cos(2.0*atan2(1.0*vz, vx)) - 2.05) - 1.0*vx*(1.2*sin(2.0*atan2(1.0*vz, vx)) + 0.2)) + 0.0003053*deltaL*omegaL^2 + 0.0003053*deltaR*omegaR^2 + 2.699e-5*omegaL*abs(omegaL) + 2.699e-5*omegaR*abs(omegaR) + 0.2652*deltaL*sign(vx)*(vx^2 + vy^2 + vz^2) + 0.2652*deltaR*sign(vx)*(vx^2 + vy^2 + vz^2)) + wn^2*wyr - 1.0*(0.2593*(vx^2 + vz^2)^(1/2)*(1.2*sin(2.0*atan2(1.0*vz, vx)) - (4.0*vz^2*sin(2.0*atan2(1.0*vz, vx)))/(vx^2 + vz^2) - (2.4*vx*vz*cos(2.0*atan2(1.0*vz, vx)))/(vx^2 + vz^2) + 0.2) + 0.06451*(vx^2 + vy^2)^(1/2)*(2.0*cos(2.0*atan2(1.0*vy, vx)) - (2.4*vy^2*cos(2.0*atan2(1.0*vy, vx)))/(vx^2 + vy^2) + (4.0*vx*vy*sin(2.0*atan2(1.0*vy, vx)))/(vx^2 + vy^2) - 2.0) + 0.5303*deltaL*vx*sign(vx) + 0.5303*deltaR*vx*sign(vx)   + (0.06451*vx*(1.2*vy*sin(2.0*atan2(1.0*vy, vx)) + vx*(2.0*cos(2.0*atan2(1.0*vy, vx)) - 2.0)))/(vx^2 + vy^2)^(1/2) + (25.93*vx*wy)/(vx^2 + vz^2)^(1/2) - (0.2593*vx*(vz*(2.0*cos(2.0*atan2(1.0*vz, vx)) - 2.05) - 1.0*vx*(1.2*sin(2.0*atan2(1.0*vz, vx)) + 0.2)))/(vx^2 + vz^2)^(1/2))*(19.64*q0*q2 - 0.06827*(vx^2 + vz^2)^(1/2)*(vx*(2.0*cos(2.0*atan2(1.0*vz, vx)) - 2.05) + vz*(1.2*sin(2.0*atan2(1.0*vz, vx)) + 0.2)) - 0.01699*(vx^2 + vy^2)^(1/2)*(1.2*vy*sin(2.0*atan2(1.0*vy, vx)) + vx*(2.0*cos(2.0*atan2(1.0*vy, vx)) - 2.0)) - 19.64*q1*q3 - 2.0*vy*wz + 2.0*vz*wy + 1.777e-6*omegaL*abs(omegaL) + 1.777e-6*omegaR*abs(omegaR) - 2.033e-5*omegaL^2 - 2.033e-5*omegaR^2 + 4.231e-7*omegaL^2*abs(deltaL) + 4.231e-7*omegaR^2*abs(deltaR) + 0.0003675*abs(deltaL)*sign(vx)*(vx^2 + vy^2 + vz^2) + 0.0003675*abs(deltaR)*sign(vx)*(vx^2 + vy^2 + vz^2));
                                                                                                                                                                                                                                                                                                                                                                                                                                                                                                                                                                                                                                                                                                                                                                                                                                                                                                                                                                              0.7763*wx*(0.06451*(vx^2 + vy^2)^(1/2)*(1.2*vy*sin(2.0*atan2(1.0*vy, vx)) + vx*(2.0*cos(2.0*atan2(1.0*vy, vx)) - 2.0)) + 25.93*wy*(vx^2 + vz^2)^(1/2) - 1.266*wx*wz - 0.2593*(vx^2 + vz^2)^(1/2)*(vz*(2.0*cos(2.0*atan2(1.0*vz, vx)) - 2.05) - 1.0*vx*(1.2*sin(2.0*atan2(1.0*vz, vx)) + 0.2)) + 0.0003053*deltaL*omegaL^2 + 0.0003053*deltaR*omegaR^2 + 2.699e-5*omegaL*abs(omegaL) + 2.699e-5*omegaR*abs(omegaR) + 0.2652*deltaL*sign(vx)*(vx^2 + vy^2 + vz^2) + 0.2652*deltaR*sign(vx)*(vx^2 + vy^2 + vz^2)) - 1.0*(0.05733*(vx^2 + vy^2)^(1/2)*(2.0 + (2.4*vx^2*cos(2.0*atan2(1.0*vy, vx)))/(vx^2 + vy^2) + (4.0*vx*vy*sin(2.0*atan2(1.0*vy, vx)))/(vx^2 + vy^2) - 2.0*cos(2.0*atan2(1.0*vy, vx))) + (0.05733*vy*(2.0*vy - 2.0*vy*cos(2.0*atan2(1.0*vy, vx)) + 1.2*vx*sin(2.0*atan2(1.0*vy, vx))))/(vx^2 + vy^2)^(1/2))*(19.64*q0*q1 - 0.01699*(vx^2 + vy^2)^(1/2)*(1.2*vx*sin(2.0*atan2(1.0*vy, vx)) - vy*(2.0*cos(2.0*atan2(1.0*vy, vx)) - 2.0)) + 19.64*q2*q3 - 2.0*vx*wz + 2.0*vz*wx) + (37.5*wz*(c44*vx^3 + c34*vx^2 + c24*vx + c14)*vz^2 + 25.0*wz*(c43*vx^3 + c33*vx^2 + c23*vx + c13)*vz + 12.5*wz*(c42*vx^3 + c32*vx^2 + c22*vx + c12))*(2.0*vy*wx - 2.0*vx*wy - 0.06827*(vx^2 + vz^2)^(1/2)*(vz*(2.0*cos(2.0*atan2(1.0*vz, vx)) - 2.05) - 1.0*vx*(1.2*sin(2.0*atan2(1.0*vz, vx)) + 0.2)) + 8.462e-6*deltaL*omegaL^2 + 8.462e-6*deltaR*omegaR^2 + 7.108e-6*omegaL*abs(omegaL) + 7.108e-6*omegaR*abs(omegaR) - 9.82*q0^2 + 9.82*q1^2 + 9.82*q2^2 - 9.82*q3^2 + 0.00735*deltaL*sign(vx)*(vx^2 + vy^2 + vz^2) + 0.00735*deltaR*sign(vx)*(vx^2 + vy^2 + vz^2)) - 0.7763*wy*(14.29*a11*wx - 0.00728*(vx^2 + vy^2)^(1/2)*(2.0*vy - 2.0*vy*cos(2.0*atan2(1.0*vy, vx)) + 1.2*vx*sin(2.0*atan2(1.0*vy, vx))) + 14.29*b11*wz - 1.03*wy*wz - 5.803e-5*deltaL*omegaL^2 + 5.803e-5*deltaR*omegaR^2 + 14.29*a31*vx^2*wx + 14.29*a41*vx^3*wx + 14.29*b31*vx^2*wz + 14.29*vz^2*wz*(b33*vx^2 + b23*vx + b13) + 14.29*vz^3*wz*(b34*vx^2 + b24*vx + b14) + 14.29*vz*wx*(a42*vx^3 + a32*vx^2 + a22*vx + a12) - 0.0504*deltaL*sign(vx)*(vx^2 + vy^2 + vz^2) + 0.0504*deltaR*sign(vx)*(vx^2 + vy^2 + vz^2) + 14.29*a21*vx*wx + 14.29*b21*vx*wz + 14.29*vz^2*wx*(a43*vx^3 + a33*vx^2 + a23*vx + a13) + 14.29*vz*wz*(b32*vx^2 + b22*vx + b12)) + 0.0002515*omegaL*(20.0*omegaL - 20.0*u_jointT) - 0.0002515*omegaR*(20.0*omegaR - 20.0*u_jointT) + (12.5*c21*wz - 0.05733*(vx^2 + vy^2)^(1/2)*(- 1.2*sin(2.0*atan2(1.0*vy, vx)) + (4.0*vy^2*sin(2.0*atan2(1.0*vy, vx)))/(vx^2 + vy^2) + (2.4*vx*vy*cos(2.0*atan2(1.0*vy, vx)))/(vx^2 + vy^2)) + 37.5*c41*vx^2*wz + 12.5*vz*wz*(3.0*c42*vx^2 + 2.0*c32*vx + c22) + (0.05733*vx*(2.0*vy - 2.0*vy*cos(2.0*atan2(1.0*vy, vx)) + 1.2*vx*sin(2.0*atan2(1.0*vy, vx))))/(vx^2 + vy^2)^(1/2) + 25.0*c31*vx*wz + 12.5*vz^2*wz*(3.0*c43*vx^2 + 2.0*c33*vx + c23) + 12.5*vz^3*wz*(3.0*c44*vx^2 + 2.0*c34*vx + c24))*(19.64*q0*q2 - 0.06827*(vx^2 + vz^2)^(1/2)*(vx*(2.0*cos(2.0*atan2(1.0*vz, vx)) - 2.05) + vz*(1.2*sin(2.0*atan2(1.0*vz, vx)) + 0.2)) - 0.01699*(vx^2 + vy^2)^(1/2)*(1.2*vy*sin(2.0*atan2(1.0*vy, vx)) + vx*(2.0*cos(2.0*atan2(1.0*vy, vx)) - 2.0)) - 19.64*q1*q3 - 2.0*vy*wz + 2.0*vz*wy + 1.777e-6*omegaL*abs(omegaL) + 1.777e-6*omegaR*abs(omegaR) - 2.033e-5*omegaL^2 - 2.033e-5*omegaR^2 + 4.231e-7*omegaL^2*abs(deltaL) + 4.231e-7*omegaR^2*abs(deltaR) + 0.0003675*abs(deltaL)*sign(vx)*(vx^2 + vy^2 + vz^2) + 0.0003675*abs(deltaR)*sign(vx)*(vx^2 + vy^2 + vz^2)) + wn^2*wz + wn^2*wzr + 2.0*wn*(0.05733*(vx^2 + vy^2)^(1/2)*(1.2*vx*sin(2.0*atan2(1.0*vy, vx)) - vy*(2.0*cos(2.0*atan2(1.0*vy, vx)) - 2.0)) + 12.5*c11*wz + 12.5*vz*(c42*wz*vx^3 + c32*wz*vx^2 + c22*wz*vx + c12*wz) + 12.5*vz^2*(c43*wz*vx^3 + c33*wz*vx^2 + c23*wz*vx + c13*wz) + 12.5*vz^3*(c44*wz*vx^3 + c34*wz*vx^2 + c24*wz*vx + c14*wz) + 0.0001258*omegaL^2 - 0.0001258*omegaR^2 + 12.5*c31*vx^2*wz + 12.5*c41*vx^3*wz + 12.5*c21*vx*wz) - 1.0*(12.5*c11 + 12.5*vz*(c42*vx^3 + c32*vx^2 + c22*vx + c12) + 12.5*c21*vx + 12.5*vz^2*(c43*vx^3 + c33*vx^2 + c23*vx + c13) + 12.5*vz^3*(c44*vx^3 + c34*vx^2 + c24*vx + c14) + 12.5*c31*vx^2 + 12.5*c41*vx^3)*(0.05733*(vx^2 + vy^2)^(1/2)*(2.0*vy - 2.0*vy*cos(2.0*atan2(1.0*vy, vx)) + 1.2*vx*sin(2.0*atan2(1.0*vy, vx))) + 12.5*c11*wz + 0.7763*wx*wy + 0.0001258*omegaL^2 - 0.0001258*omegaR^2 + 12.5*c31*vx^2*wz + 12.5*c41*vx^3*wz + 12.5*vz*wz*(c42*vx^3 + c32*vx^2 + c22*vx + c12) + 12.5*c21*vx*wz + 12.5*vz^2*wz*(c43*vx^3 + c33*vx^2 + c23*vx + c13) + 12.5*vz^3*wz*(c44*vx^3 + c34*vx^2 + c24*vx + c14)) ...
];
%

u_ref = M\K;

cond_M = cond(M);

u_deltaA = u_ref(1);
u_jointA = u_ref(2);
u_deltaT = u_ref(3);

u_deltaL = u_jointA - u_deltaA/2;
u_deltaR = u_jointA + u_deltaA/2;
u_omegaL = u_jointT + u_deltaT/2;
u_omegaR = u_jointT - u_deltaT/2;

end

== matlab function TailSitter_PX4/q_fly_generator/MATLAB Function3 ==
  data: pitchPID input; vherror output; pitch output; vr_wf input; v_wf input
function [vherror,pitch] = setpitch(pitchPID,vr_wf, v_wf)

pitch = 0;

% Angle toward horizon given by:
horzspeedr = sqrt(sum(vr_wf(1:2).^2));  % Horizontal speed requested
pitch = (horzspeedr +6.013)/15.38;      % From simulations and linefitting
pitch = (pi/2-pitch);                   % correct for coordsys

% We can choose:
%   - Regulate horizontal speed with pitch and altitude with engine power
%   - Regulate horizontal speed with engine power and altitude with pitch.
%
% The first option makes sense when hovering but may be problematic when
% flying: if we are horizontally oriented and dropping in altitude engine
% power cannot do anything about it. However, it will try to increase speed
% forcing the pitch controller to pitch up to reduce speed. Might work.
% The second option makes sense when flying. When hovering we have no
% horizontal speed though.
%

horzspeed  = sqrt(sum( v_wf(1:2).^2));  % Actual horizontal speed
vherror = horzspeedr-horzspeed;         % Error in horizontal speed, to be
                                        % sent to externa PID.

% correct pitch using measurments, use external pid
pitch = pitch + pitchPID;


% use error in direction to roll slightly, use external PID
%roll = 0.1*yawe;

== matlab function TailSitter_PX4/MATLAB Function9 ==
  data: q_fly input; vr_wf input; v_cutoff input; q_ref output; q_hover input; hovermode output
function [q_ref, hovermode] = modeswitcher(q_fly, vr_wf, v_cutoff, q_hover)

hspeed = sqrt(sum( vr_wf(1:2).^2 ));
vspeed = abs(vr_wf(3));

Theta = atan2(hspeed, vspeed);

rspeed = sqrt(sum( vr_wf.^2 ));
if rspeed < v_cutoff || abs(Theta) < deg2rad(20)
    q_ref = q_hover;
    hovermode = 1;
else
    q_ref = q_fly;
    hovermode=0;
end

== matlab function TailSitter_PX4/linegenerator1 ==
  settings: updateMethod=DISCRETE
  data: max2l input; d2lcoeff input; r input; altError output; p parameter; rspeed output; refvec output; wpN output; dist2wp output; vec2line output
function [altError, rspeed, refvec, wpN, dist2wp, vec2line] = LineGenerator(max2l, d2lcoeff ,r,p)

% Keep track of which waypoint we are going to
persistent waypointno;
persistent wp;
persistent wp_prev;
if isempty(waypointno)
    waypointno = 1;
    wp = p.waypoints(waypointno,:)';
    wp_prev = p.waypoints(waypointno,:)';
end

%initialize variables
dist2line2d = 0;
altError = 0;
rspeed = 0;
vec2line = [0,0,0]';

% if current waypoint is the start wp/home wp jump immediately to next.
dist2wp = sqrt( sum( (wp(1:3)-r).^2 ) );
if dist2wp <= p.wpradius
    if waypointno < p.numwp
        waypointno = waypointno+1;
    else
        waypointno = 1; 
    end
    wp_prev = wp;
    wp = p.waypoints(waypointno,:)';
end
rspeed = wp(4);

% find vector between last waypoint and current target
linevec = (wp(1:3)-wp_prev(1:3))./sqrt( sum((wp(1:3)-wp_prev(1:3)).^2) );

% Figure out if goal is ahead of us or if we passed it/missed it.
%if dot(v_wf(1:3), wp(1:3)-r(1:3)) < 0
%    linevec(1:2) = - linevec(1:2);
%end
% THe above doesn't work.


% Find the vector that describes the vector to the closest point on the
% line
a = wp_prev(1:3);
n = linevec;
vec2line = a-r - dot(a-r,n)*n;
altError = vec2line(3);
dist2line2d = sqrt( sum( vec2line(1:2).^2 ));
wpN = waypointno;


% Mix the vectors for reference according to how far away from line we are
%cr = cross(linevec,vec2line);
%refvec = linevec;
if abs(d2lcoeff*dist2line2d) < max2l
    refvec = linevec + d2lcoeff*dist2line2d*vec2line;
else
    refvec = linevec + max2l*vec2line;
end
refvec = refvec/sqrt(sum(refvec.^2));

== matlab function TailSitter_PX4/q_fly_generator/ZYX-quat ==
  data: y input; z input; q output; x input
function q = rotang2quat(y,z,x)

q = [0,0,0,0];

u = [z,y,x];
qa = quaternion(u, 'euler', 'ZYX', 'frame');
q = qa.compact;

== matlab function TailSitter_PX4/q_fly_generator/MATLAB Function5 ==
  data: yawr input; yaw input; yawe output
function yawe = fcn(yawr,yaw)

% IF our angle error is more than 180 degrees we need to cross the sign
% barrier, this code should take care of that.
% Since rate limiters are in play, we might need to loo at yawr_target, but
% lets wait with that for now.

yawe = yawr-yaw;
% r:100, y:-90 => e=190 => -360+190= -170
% r:-100, y=90 => e=-190 => 360+(-190) = 170
if yawe > pi
    yawe = -2*pi+yawe;
elseif yawe < -pi
    yawe = 2*pi+yawe;
end

== matlab function TailSitter_PX4/q_fly_generator/MATLAB Function6 ==
  data: yawr input; maxrate input; yawr_last input; yawr_slow output; p parameter
function yawr_slow  = fcn(yawr, maxrate, yawr_last, p)

%This is a rate limiter that takes into account which direction is closest
%to the reference, i.e. makes sure we cross the sign at +-pi if we need to.

% We would like to set yawr_slow to yawr, but can only approach it in steps
% of maxrate.
yawr_slow = yawr;
e = yawr-yawr_last;
% slew rate = unit/s => (unit*sampletime)/s
maxrate = maxrate*p.Ts;

if abs(e) > maxrate
    if e > pi
        yawr_slow = yawr_last - maxrate;
    elseif e < -pi
        yawr_slow = yawr_last + maxrate;
    else
        yawr_slow = yawr_last + sign(e)*maxrate;
    end
end

while(yawr_slow > pi)
    yawr_slow = yawr_slow - 2*pi;
end
while(yawr_slow < -pi)
    yawr_slow = yawr_slow + 2*pi;
end

end

== matlab function TailSitter_PX4/MATLAB Function7 ==
  data: refvec input; qref output
function qref = refvec2refquat(refvec)

qref = [0,0,0,0];

% set yaw correct
if sqrt(sum( refvec(1:2).^2 )) < 0.1 % Check if we are only pointing up
    Y = 0;
else
    Y = atan2(refvec(2),refvec(1));
end
qY = [cos(Y/2),0,0,sin(Y/2)];

% set pitch correct
hspeed = sqrt(sum(refvec(1:2)).^2);
T = atan2(refvec(3),hspeed);
qT = [cos(T/2),0,sin(T/2),0];


% Set roll to horizontal
qR = [1,0,0,0];

qref = quatmultiply(quatmultiply(qY,qT), qR);

== matlab function TailSitter_PX4/q_fly_generator/MATLAB Function8 ==
  data: vr_wf input; yawr output; v_wf input; yaw output
function [yawr,yaw] = setyaw(vr_wf,v_wf)

% reference heading
yawr = atan2(vr_wf(2),vr_wf(1));
%current heading
 yaw = atan2(v_wf(2),v_wf(1));

== matlab function TailSitter_PX4/FlyVecAdjust ==
  data: rspeed input; refvec output; vec2line input; linevec input; d2lcoeff input
function refvec = flyVecAdjust(rspeed, vec2line,linevec, d2lcoeff)

vcomp=1/rspeed;
refvec = linevec+vec2line*d2lcoeff*vcomp;

refvec = refvec/sqrt(sum(refvec.^2));

== matlab function TailSitter_PX4/MATLAB Function11 ==
  data: axisgains input; angErr input; taos output; w input
function taos = taos_fordecoupler(axisgains,angErr, w)

taos = [0;0;0];

P1 = 30; %1
P2 = 7.5; %0.25
cx = axisgains(1);%10;
cy = axisgains(2);%100;
cz = axisgains(3);%1;


% Emil Fresk P2 controller
taos = -P1.*angErr - P2.*w;
% Adjustment for actuators
taos(1) = cx*taos(1);
taos(2) = cy*taos(2);
taos(3) = cz*taos(3);

== matlab function TailSitter_PX4/MATLAB Function12 ==
  data: hovermode input; c output; c_hov input; max_hov input; c_fly input; max_fly input; max output
function [c, max] = fcn(hovermode, c_hov, max_hov, c_fly, max_fly)

if hovermode
    c = c_hov;
    max = max_hov;
else
    c = c_fly;
    max = max_fly;
end
